simulink model "fresh_control_system"  (R2020a)
settings: Solver=VariableStepAuto  StartTime=0.0  StopTime=7  RelTol=1e-3
libraries: simulink x2, dspfdesign x1
settings Model: Creator=parthmahendru  LastModifiedBy=Mohamed
settings OptimizationCC: DefaultParameterBehavior=Inlined  EnhancedBackFolding=on  PassReuseOutputArgsAs=Individual arguments  ZeroExternalMemoryAtStartup=off  ZeroInternalMemoryAtStartup=off  OptimizeBlockOrder=speed  DifferentSizesBufferReuse=on  EfficientTunableParamExpr=on
settings DebuggingCC: ParameterTunabilityLossMsg=error
settings SFSimCC: MATLABDynamicMemAlloc=off
settings RTWCC: SystemTargetFile=ert.tlc  GenCodeOnly=on  TemplateMakefile=ert_default_tmf
settings CodeAppCC: ForceParamTrailComments=on  IgnoreCustomStorageClasses=off  OperatorAnnotations=on  SimulinkDataObjDesc=on  SFDataObjDesc=on  InsertBlockDesc=on
settings ERTTargetCC: TargetLangStandard=C99 (ISO)  GenerateSampleERTMain=on  InlinedParameterPlacement=NonHierarchical  ERTCustomFileTemplate=example_file_process.tlc

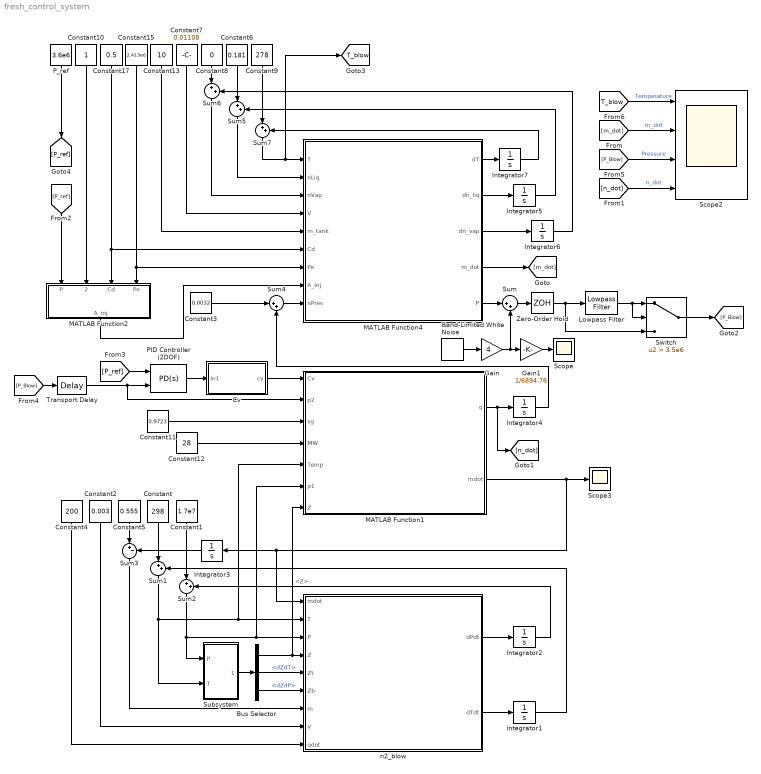
== system fresh_control_system ==
  Band-Limited White Noise : simulink/Sources/Band-Limited White Noise  Cov=100000  Ts=0.001  seed=[23341]
  Bus Selector : BusSelector  OutputSignals=Z,dZdT,dZdP
  Constant : Constant  Value=298
  Constant1 : Constant  Value=1.7e7
  Constant10 : Constant
  Constant11 : Constant  Value=0.9723
  Constant12 : Constant  Value=28
  Constant13 : Constant  Value=10
  Constant15 : Constant  Value=2.413e6  VectorParams1D=off
  Constant17 : Constant  Value=0.5
  Constant2 : Constant  Value=0.003
  Constant3 : Constant  Value=0.0032
  Constant4 : Constant  Value=200
  Constant5 : Constant  Value=0.555
  Constant6 : Constant  Value=0.181
  Constant7 : Constant  Value=0.01108
  Constant8 : Constant  Value=0
  Constant9 : Constant  Value=278
  Cv : Subsystem
  Gain : Gain  Gain=4
  Gain1 : Gain  Gain=1/6894.76
  Integrator{1..7} (7 alike) : Integrator
  Lowpass Filter : dspfdesign/Lowpass Filter  FilterType=FIR  DesignForMinimumOrder=off  FilterOrder=10  PassbandFrequency=700  StopbandFrequency=3000  PassbandRipple=0.1  StopbandAttenuation=80  InheritSampleRate=off  SampleRate=44100  SimulateUsing=Interpreted execution  roundingMode=Nearest  coeffsDataTypeStr=fixdt(1,16)
  MATLAB Function1 : MATLAB Function  TreatAsAtomicUnit=on
  MATLAB Function2 : MATLAB Function  TreatAsAtomicUnit=on
  MATLAB Function4 : MATLAB Function  TreatAsAtomicUnit=on
  PID Controller (2DOF) : simulink/Continuous/PID Controller (2DOF)  Controller=PD  Form=Parallel  TimeDomain=Continuous-time  UseExternalTs=off  SampleTime=-1  IntegratorMethod=Forward Euler  FilterMethod=Forward Euler  ControllerParametersSource=internal  P=3.2e-09  I=1.39281882332403e-13  D=0.9e-05  UseFilter=on  N=1.09398371936337  b=1  c=1  TunerSelectOption=Transfer Function Based (PID Tuner App)  InitialConditionSource=internal  InitialConditionForIntegrator=0  InitialConditionForFilter=0  DifferentiatorICPrevScaledInput=0  ExternalReset=none  TrackingMode=off  Kt=1  LimitOutput=on  UpperSaturationLimit=5  LowerSaturationLimit=0  LinearizeAsGain=on  AntiWindupMode=none  Kb=1  POutMin=[]  POutMax=[]  IOutMin=[]  IOutMax=[]  DOutMin=[]  DOutMax=[]  NOutMin=[]  NOutMax=[]  bOutMin=[]  bOutMax=[]  cOutMin=[]  cOutMax=[]  SumOutMin=[]  SumOutMax=[]  SaturationOutMin=[]  SaturationOutMax=[]  PParamMin=[]  PParamMax=[]  IParamMin=[]  IParamMax=[]  DParamMin=[]  DParamMax=[]  NParamMin=[]  NParamMax=[]  bParamMin=[]  bParamMax=[]  cParamMin=[]  cParamMax=[]  KbParamMin=[]  KbParamMax=[]  KtParamMin=[]  KtParamMax=[]  KbOutMin=[]  KbOutMax=[]  KtOutMin=[]  KtOutMax=[]  IntegratorOutMin=[]  IntegratorOutMax=[]  FilterOutMin=[]  FilterOutMax=[]  SumI1OutMin=[]  SumI1OutMax=[]  SumI2OutMin=[]  SumI2OutMax=[]  SumI3OutMin=[]  SumI3OutMax=[]  SumI4OutMin=[]  SumI4OutMax=[]  SumDOutMin=[]  SumDOutMax=[]  Sum1OutMin=[]  Sum1OutMax=[]  Sum2OutMin=[]  Sum2OutMax=[]  Sum3OutMin=[]  Sum3OutMax=[]  DifferentiatorOutMin=[]  DifferentiatorOutMax=[]  FilterDiffOutCoefMin=[]  FilterDiffOutCoefMax=[]  ReciprocalOutMin=[]  ReciprocalOutMax=[]  SumDenOutMin=[]  SumDenOutMax=[]  SumNumOutMin=[]  SumNumOutMax=[]  DivideOutMin=[]  DivideOutMax=[]  UdiffTsProdOutMin=[]  UdiffTsProdOutMax=[]  NTsProdOutMin=[]  NTsProdOutMax=[]  UintegralTsProdOutMin=[]  UintegralTsProdOutMax=[]  UngainTsProdOutMin=[]  UngainTsProdOutMax=[]  IntegratorContinuousStateAttributes=''  IntegratorStateMustResolveToSignalObject=off  IntegratorRTWStateStorageClass=Auto  FilterContinuousStateAttributes=''  FilterStateMustResolveToSignalObject=off  FilterRTWStateStorageClass=Auto  ParallelPVariant=InternalParameters  IdealPVariant=Disabled  IVariant=Disabled  DVariant=InternalParameters  bVariant=InternalParameters  cVariant=InternalParameters  IntegratorVariant=Disabled  SatVariant=Enabled  AWVariant=Disabled  PCopyVariant=Disabled  TRVariant=Disabled  FdbkBlocksVariant=Forward  IdealPFdbkVariant=Disabled  SatFdbkVariant=Disabled  DerivativeFilterVariant=ContFilter  NVariant=InternalParameters  NCopyVariant=Disabled  FilterICVariant=InternalICsFilter  IntegratorICVariant=Disabled  ExternalResetVariant=Disabled  TRSumVariant=Passthrough  SumFdbkVariant=Disabled  SumVariant=Sum_PD  TsampFilterVariant=InternalTs  TsampNgainVariant=Passthrough  TsampIntegralVariant=Disabled_SignalSpec
  P_ref : Constant  Value=3.6e6
  Scope : Scope
  Scope2 : Scope  NumInputPorts=4
  Scope3 : Scope
  Subsystem : Subsystem
  Sum{,1..2,4..7} (7 alike) : Sum  Inputs=|++
  Sum3 : Sum  Inputs=|+-
  Switch : Switch  Criteria=u2 > Threshold  Threshold=3.5e6
  Transport Delay : TransportDelay  DelayTime=0.01
  Zero-Order Hold : ZeroOrderHold  SampleTime=-1
  n2_blow : MATLAB Function  TreatAsAtomicUnit=on
  tag scope: T_blow=global
  wires:
  PID Controller (2DOF)/1 -> Cv/1(In1)
  MATLAB Function4/4(m_dot) -> [m_dot]
  [m_dot] -> Scope2/2  "m_dot"
  [n_dot] -> Scope2/4  "n_dot"
  [P_Blow] -> Scope2/3  "Pressure"
  [T_blow] -> Scope2/1  "Temperature"
  Constant4/1 -> n2_blow/9(qdot)
  Constant2/1 -> n2_blow/8(V)
  Constant1/1 -> Sum2/1
  n2_blow/1(dPdt) -> Integrator2/1
  Integrator2/1 -> Sum2/2
  Integrator1/1 -> Sum1/2
  n2_blow/2(dTdt) -> Integrator1/1
  Constant/1 -> Sum1/1
  Constant5/1 -> Sum3/1
  Sum3/1 -> n2_blow/7(m)
  MATLAB Function1/2(mdot) -> Scope3/1, n2_blow/1(mdot), Integrator3/1
  Integrator3/1 -> Sum3/2
  Sum4/1 -> MATLAB Function4/9(nPres)
  Constant3/1 -> Sum4/1
  Constant6/1 -> Sum5/1
  MATLAB Function4/1(dT) -> Integrator7/1
  MATLAB Function4/2(dn_liq) -> Integrator5/1
  MATLAB Function4/3(dn_vap) -> Integrator6/1
  Sum5/1 -> MATLAB Function4/2(nLiq)
  Integrator5/1 -> Sum5/2
  Constant8/1 -> Sum6/1
  Sum6/1 -> MATLAB Function4/3(nVap)
  Integrator6/1 -> Sum6/2
  Constant9/1 -> Sum7/1
  Integrator7/1 -> Sum7/2
  Sum7/1 -> [T_blow], MATLAB Function4/1(T)
  MATLAB Function1/1(q) -> [n_dot], Integrator4/1
  Integrator4/1 -> Sum4/2
  Constant7/1 -> MATLAB Function4/4(V)
  Constant13/1 -> MATLAB Function4/5(m_tank)
  Constant15/1 -> MATLAB Function2/4(Pe), MATLAB Function4/7(Pe)
  Constant17/1 -> MATLAB Function2/3(Cd), MATLAB Function4/6(Cd)
  MATLAB Function2/1(A_inj) -> MATLAB Function4/8(A_inj)
  Constant10/1 -> MATLAB Function2/2(m_dot_des)
  P_ref/1 -> [P_ref]
  [P_ref] -> MATLAB Function2/1(P)
  MATLAB Function4/5(P) -> Sum/1
  Band-Limited White Noise/1 -> Gain/1
  [P_ref] -> PID Controller (2DOF)/1
  [P_Blow] -> Transport Delay/1
  Sum/1 -> Zero-Order Hold/1
  Zero-Order Hold/1 -> Lowpass Filter/1, Switch/3
  Gain/1 -> Sum/2, Gain1/1
  Switch/1 -> [P_Blow]
  Lowpass Filter/1 -> Switch/2, Switch/1
  Gain1/1 -> Scope/1
  Sum2/1 -> MATLAB Function1/6(p1), n2_blow/3(P), Subsystem/1(P)
  Sum1/1 -> MATLAB Function1/5(Temp), n2_blow/2(T), Subsystem/2(T)
  Subsystem/1(Outport) -> Bus Selector/1
  Bus Selector/2 -> n2_blow/5(Zt)  "<dZdT>"
  Bus Selector/3 -> n2_blow/6(Zb)  "<dZdP>"
  Bus Selector/1 -> MATLAB Function1/7(Z), n2_blow/4(Z)  "<Z>"
  Constant11/1 -> MATLAB Function1/3(sg)
  Constant12/1 -> MATLAB Function1/4(MW)
  Transport Delay/1 -> MATLAB Function1/2(p2), PID Controller (2DOF)/2
  Cv/1(cv) -> MATLAB Function1/1(Cv)

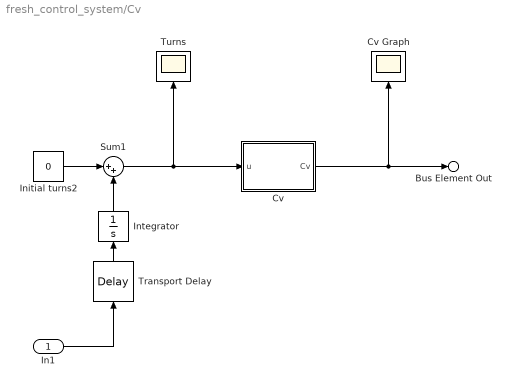
== system fresh_control_system/Cv ==
  In1 : Inport
  Cv : MATLAB Function  TreatAsAtomicUnit=on
  Cv Graph : Scope
  Initial turns2 : Constant  Value=0
  Integrator : Integrator
  Sum1 : Sum  Inputs=|++
  Transport Delay : TransportDelay  DelayTime=0.004
  Turns : Scope
  Bus Element Out : Outport  PortName=cv  Element=signal1
  wires:
  In1/1 -> Transport Delay/1
  Integrator/1 -> Sum1/2
  Initial turns2/1 -> Sum1/1
  Cv/1(Cv) -> Cv Graph/1, Bus Element Out/1
  Sum1/1 -> Cv/1(u), Turns/1
  Transport Delay/1 -> Integrator/1

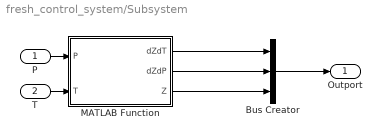
== system fresh_control_system/Subsystem ==
  P : Inport
  T : Inport  Port=2
  Bus Creator : BusCreator  Inputs=3
  MATLAB Function : MATLAB Function  TreatAsAtomicUnit=on
  Outport : Outport
  wires:
  MATLAB Function/1(dZdT) -> Bus Creator/1
  T/1 -> MATLAB Function/2(T)
  MATLAB Function/2(dZdP) -> Bus Creator/2
  P/1 -> MATLAB Function/1(P)
  MATLAB Function/3(Z) -> Bus Creator/3
  Bus Creator/1 -> Outport/1

== matlab function fresh_control_system/MATLAB Function2 ==
  data: P input; A_inj output; m_dot_des input; Cd input; Pe input
function A_inj  = A_inj(P, m_dot_des, Cd, Pe)
MW=44;
Vhat_l=0.05;

A_inj=(m_dot_des)/(Cd*sqrt(abs(2/MW*(P - Pe)/Vhat_l))*MW);

== matlab function fresh_control_system/n2_blow ==
  data: mdot input; T input; P input; Z input; Zt input; Zb input; m input; V input; dPdt output; qdot input; dTdt output
function [dPdt, dTdt] = n2_blowdown(mdot, T, P, Z, Zt, Zb, m, V, qdot)

    R = 8314 / 28;
    cnv = 6894.76;

    Zp = Zb/cnv;
    cv = 776;

    dPdt = (m*R*Z^2 + P*V*Zt)*qdot/(V*cv*(m*(Z - P*Zp)))    ...
         - mdot*((cv + Z*R)*m*Z + P*V*Zt)*(P/(m*cv))/(m*(Z - P*Zp));

    dZdt = (m*R*Z^2 * Zp + V*Z*Zt)*dPdt/(m*R*Z^2 + P*V)     ...
         - Zt*(P*V*Z/m)*mdot/(m*R*Z^2 + P*V);

    dTdt = V*(dPdt/(m*Z) - dZdt*P/(m*Z^2) - mdot*P/(m*Z^2))/R;
end

== matlab function fresh_control_system/Subsystem/MATLAB Function ==
  data: P input; T input; dZdT output; dZdP output; Z output
function [dZdT, dZdP, Z]  = get_dZ_N2(P, T)

    P           = P / 6894.76;
    
    nh_theta    = [0.90370032155133;...
                          -3.99164830787538;...
                           4.44554878990612;...
                          -1.68387394930366;...
                           1.84282855081908;...
                          -2.71807522455834;...
                           1.80658523674363;...
                          -0.00026662830718;...
                           0.16405364316350];

    nh_alpha    = [1;               ...
                           0.45607085009281;...
                           0.99224794564113;...
                           1.58495789262624;...
                           0.53133147588636;...
                           1.29132167947510;...
                           1.44008913900161;...
                           2.74997487910292;...
                           2.36611999082672];

    nl_theta    = [0.46742656471647;...
                          -0.53799565472298;...
                          -9.22454428760102;...
                           9.15603503101003;...
                           3.18808664459882;...
                           0.30163700042055;...
                          -0.27300234680706;...
                          -1.00749719408221;...
                          -1.49106816983329];

    nl_alpha    = [1;               ...
                           1.41102397459172;...
                           0.33562799290636;...
                           0.79810083070486;...
                           0.01008992455881;...
                           2.53968667359886;...
                           2.51281397715323;...
                           1.20879498088509;...
                           1.69572064361084];
                       
    if (T >= 220 && T <= 320) && (P >= 800 && P <= 4500)

        T           = T / 126.2;
        P           = P / 492.3;

        dZdTr       = nh_theta(2)*nh_alpha(2)*T^(nh_alpha(2) - 1)*P^0.7   ...
                    + nh_theta(3)*nh_alpha(3)*T^(nh_alpha(3) - 1)*P^0.5   ...
                    + nh_theta(4)*nh_alpha(4)*T^(nh_alpha(4) - 1)*P^0.3   ...
                    + nh_theta(5)*nh_alpha(5)*T^(nh_alpha(5) - 1)*P       ...
                    + nh_theta(6)*nh_alpha(6)*T^(nh_alpha(6) - 1)*P       ...
                    + nh_theta(7)*nh_alpha(7)*T^(nh_alpha(7) - 1)*P       ...
                    + nh_theta(9)*nh_alpha(9)*T^(nh_alpha(9) - 1);

        dZdT        = dZdTr / 126.2;

        dZdPr       = 0.7*nh_theta(2)*T^nh_alpha(2)*P^(-0.3)        ...
                    + 0.5*nh_theta(3)*T^nh_alpha(3)*P^(-0.5)        ...
                    + 0.3*nh_theta(4)*T^nh_alpha(4)*P^(-0.7)        ...
                    + nh_theta(5)*T^nh_alpha(5)                     ...
                    + nh_theta(6)*T^nh_alpha(6)                     ...
                    + nh_theta(7)*T^nh_alpha(7)                     ...
                    + nh_theta(8)*nh_alpha(8)*P^(nh_alpha(8) - 1);

        dZdP        = dZdPr / 492.3;     

        N           = [1;                       ...
                        T^nh_alpha(2)*P^0.7;     ...
                        T^nh_alpha(3)*P^0.5;     ...
                        T^nh_alpha(4)*P^0.3;     ...
                        T^nh_alpha(5)*P;           ...
                        T^nh_alpha(6)*P;           ...
                        T^nh_alpha(7)*P;           ...
                        P^nh_alpha(8);             ...
                        T^nh_alpha(9)];               

        Z       = sum(nh_theta .* N);        

    elseif (T >= 180 && T < 220) && (P >= 800 && P <= 4500)

        T           = T / 126.2;
        P           = P / 492.3;

        dZdTr       = nl_theta(2)*nl_alpha(2)*T^(nl_alpha(2) - 1)*P^0.7   ...
                    + nl_theta(3)*nl_alpha(3)*T^(nl_alpha(3) - 1)*P^0.5   ...
                    + nl_theta(4)*nl_alpha(4)*T^(nl_alpha(4) - 1)*P^0.3   ...
                    + nl_theta(5)*nl_alpha(5)*T^(nl_alpha(5) - 1)*P       ...
                    + nl_theta(6)*nl_alpha(6)*T^(nl_alpha(6) - 1)*P       ...
                    + nl_theta(7)*nl_alpha(7)*T^(nl_alpha(7) - 1)*P       ...
                    + nl_theta(9)*nl_alpha(9)*T^(nl_alpha(9) - 1);

        dZdT        = dZdTr / 126.2;

        dZdPr       = 0.7*nl_theta(2)*T^nl_alpha(2)*P^(-0.3)        ...
                    + 0.5*nl_theta(3)*T^nl_alpha(3)*P^(-0.5)        ...
                    + 0.3*nl_theta(4)*T^nl_alpha(4)*P^(-0.7)        ...
                    + nl_theta(5)*T^nl_alpha(5)                     ...
                    + nl_theta(6)*T^nl_alpha(6)                     ...
                    + nl_theta(7)*T^nl_alpha(7)                     ...
                    + nl_theta(8)*nl_alpha(8)*P^(nl_alpha(8) - 1);

        dZdP        = dZdPr / 492.3;     

        N           = [1;                       ...
                        T^nl_alpha(2)*P^0.7;     ...
                        T^nl_alpha(3)*P^0.5;     ...
                        T^nl_alpha(4)*P^0.3;     ...
                        T^nl_alpha(5)*P;           ...
                        T^nl_alpha(6)*P;           ...
                        T^nl_alpha(7)*P;           ...
                        P^nl_alpha(8);             ...
                        T^nl_alpha(9)];               

        Z       = sum(nl_theta .* N); 

    else
        T           = 180 / 126.2;
        P           = P / 492.3;

        dZdTr       = nl_theta(2)*nl_alpha(2)*T^(nl_alpha(2) - 1)*P^0.7   ...
                    + nl_theta(3)*nl_alpha(3)*T^(nl_alpha(3) - 1)*P^0.5   ...
                    + nl_theta(4)*nl_alpha(4)*T^(nl_alpha(4) - 1)*P^0.3   ...
                    + nl_theta(5)*nl_alpha(5)*T^(nl_alpha(5) - 1)*P       ...
                    + nl_theta(6)*nl_alpha(6)*T^(nl_alpha(6) - 1)*P       ...
                    + nl_theta(7)*nl_alpha(7)*T^(nl_alpha(7) - 1)*P       ...
                    + nl_theta(9)*nl_alpha(9)*T^(nl_alpha(9) - 1);

        dZdT        = dZdTr / 126.2;

        dZdPr       = 0.7*nl_theta(2)*T^nl_alpha(2)*P^(-0.3)        ...
                    + 0.5*nl_theta(3)*T^nl_alpha(3)*P^(-0.5)        ...
                    + 0.3*nl_theta(4)*T^nl_alpha(4)*P^(-0.7)        ...
                    + nl_theta(5)*T^nl_alpha(5)                     ...
                    + nl_theta(6)*T^nl_alpha(6)                     ...
                    + nl_theta(7)*T^nl_alpha(7)                     ...
                    + nl_theta(8)*nl_alpha(8)*P^(nl_alpha(8) - 1);

        dZdP        = dZdPr / 492.3;  

    N           = [1;                       ...
                    T^nl_alpha(2)*P^0.7;     ...
                    T^nl_alpha(3)*P^0.5;     ...
                    T^nl_alpha(4)*P^0.3;     ...
                    T^nl_alpha(5)*P;           ...
                    T^nl_alpha(6)*P;           ...
                    T^nl_alpha(7)*P;           ...
                    P^nl_alpha(8);             ...
                    T^nl_alpha(9)];               

    Z       = sum(nl_theta .* N); 

    end
end

== matlab function fresh_control_system/MATLAB Function4 ==
  data: T input; dT output; dn_liq output; dn_vap output; m_dot output; nLiq input; nVap input; V input; m_tank input; Cd input; Pe input; A_inj input; P output; nPres input
function [dT, dn_liq, dn_vap, m_dot, P] = nox_blowdown(T, nLiq, nVap, V, m_tank, Cd, Pe, A_inj, nPres )
%OX_TANK_SIM Models thermochemical processes of blow-down in oxidizer tank.
%   Propellant Tank Pressurization Modeling for a Hybrid Rocket - Margaret
%   Mary Fernandez
%
%   INPUTS:
%       "n" = 1x2 vector of ox moles in tank (kmol).
%       "T" = ox tank temperature (K).
%       "V" = volume of ox tank (m^3).
%       "m_tank" = mass of oxidizer tank (kg).
%       "m_dot_prev" = ox mass flow rate of previous time step (kg/s).
%       "A_inj" = total orifice area of injector plate (m^2).
%       "Cd" = injector plate discharge coefficient.
%       "Pe" = pressure at exit of injector plate (Pa).
%
%   OUTPUTS:
%       "m_dot" = scalar ox mass flow rate (kg/s).
%       "dn" = 1x2 differential change in ox moles (kmol).
%       "dT" = differential change in ox tank temperature (K).
%       "P" = scalar internal pressure of ox tank (Pa).
%%%%%%%%%%%%%%%%%%%%%%%%%%%%%%%%%%%%%%%%%%%%%%%%%%%%%%%%%%%%%%%%%%%%%%%%%%%

%Perry's Chemical Engineers' Handbook Property Equations:
G1 = 96.512;           %Vapour pressure of N2O [Pa] coefficients
G2 = -4045;            % valid for Temp range [182.3 K - 309.57 K]
G3 = -12.277;
G4 = 2.886e-5;
G5 = 2;

Tc = 309.57;           % critical temperature of N2O [K]

J1 = 2.3215e7;         % heat of vaporization of N2O [J/kmol] coefficients
J2 = 0.384;            % valid for Temp range [182.3 K - 309.57 K]
J3 = 0;
J4 = 0;

% % heat capacity of N2 at constant pressure [J/(kmol*K)] coefficients
% % valid for Temp range [100 K - 1500 K]
% C1 = 0.28883e5; 
% C2 = 0;              
% C3 = 0;
% C4 = 0;
% C5 = 0;

D1 = 0.2934e5; % heat capacity of N2O gas at constant pressure [J/(kmol*K)] coefficients
D2 = 0.3236e5; % valid for Temp range [100 K - 1500 K]
D3 = 1.1238e3;
D4 = 0.2177e5;
D5 = 479.4; 

E1 = 6.7556e4; % heat capacity of N2O liquid at constant pressure [J/(kmol*K)] coefficients
E2 = 5.4373e1; % valid for Temp range [182.3 K - 200 K]
E3 = 0;
E4 = 0;
E5 = 0;
Q1 = 2.781;    % molar specific volume of liquid N2O [m^3/kmol] coefficients
Q2 = 0.27244;
Q3 = 309.57;
Q4 = 0.2882;

R  = 8314;      %Universal gas constant (J/kmol*K).
MW = 44.013;   %Molar mass of N2O (kg/kmol)​
% Calculate thermodynamic parameters as functions of temperature:
Vhat_l      = Q2^(1 + (1 - T/Q3)^Q4)/Q1;                    %Molar specific vol. of liq. N2O [m^3/kmol]
CVhat_g     = D1 + D2*((D3/T)/sinh(D3/T))^2 + ...
              D4*((D5/T)/cosh(D5/T))^2 - R;                 %Molar c_V of N2O gas [J/(kmol*K)]
CVhat_l     = E1 + E2*T + E3*T^2 + E4*T^3 + E5*T^4;         %Molar c_V of N2O liq.; approx. = c_P [J/(kmol*K)]
Tr          = T/Tc;                                         %Reduced temperature.
delta_Hv    = J1*(1 - Tr) ^ (J2 + J3*Tr + J4*Tr^2);         %Heat of vaporization of N2O [J/kmol]
P_sat       = exp(G1 + G2/T + G3*log(T) + G4*T^G5);         %Vapour P of N20 (Pa).
dP_sat      = (-G2/(T^2) + G3/T + G4*G5*T^(G5-1)) ...       %Derivative of vapour P with respect to T.
              * exp(G1 + G2/T + G3*log(T) + G4*T^G5);        
c_P         = (4.8 + 0.00322*T)*155.239;                    %Specific heat of tank, Aluminum [J/kg*K]


%Simplified expression definitions for solution:
P = (nPres+nVap)*R*T/(V - nLiq*Vhat_l);
a = m_tank*c_P  + nPres*CVhat_l+nVap*CVhat_g + nLiq*CVhat_l;
RT = P*Vhat_l;
e = -delta_Hv + R*T;
f = -Cd*A_inj*sqrt(abs(2/MW*(P - Pe)/Vhat_l));
j = -Vhat_l*P_sat;
k = (V - nLiq*Vhat_l)*dP_sat;
l = R*T;
q = R*nVap;
Z = (-f*(-j*a + (q - k)*RT))/(a*(l + j) + (q - k)*(e - RT));
W = (-Z*(l*a + (q - k)*e))/(-j*a + (q - k)*RT);
%Time derivative of tank conditions
m_dot = -f*MW;          % Mass flow rate
dn_liq    = W;    % Time derivative of nitrous amount
dn_vap=Z;
dT    = (RT*W + e*Z)/a;  % Time derivative of tank temperature

end

== matlab function fresh_control_system/Cv/Cv ==
  data: Cv output; u input
function Cv = Cvcalc(u)
Cv = u/20;

% if (u<2)
%     Cv = u/20;
% % elseif(u>6&&u<9)
% % Cv=((1.1169*(u-5.95)^2))/100+0.03;
% else
%   Cv=0;
%     
% end
% 
%     
% % till 0.1
end

== matlab function fresh_control_system/MATLAB Function1 ==
  data: Cv input; p2 input; sg input; MW input; Temp input; p1 input; q output; mdot output; Z input
function [q, mdot]   = Needle_valve(Cv,p2,sg,MW,Temp,p1,Z)
    %sg is specific gravity
    
    p1_new=p1/98066.5;
    p2_new=p2/98066.5;

    del_p=p1_new-p2_new;
    
    R = 8314 / 28;
    rho = p1 / (R * Z * Temp);

    if (p2>0.5*p1)
        q=0.11362272*Cv*p1_new*(1-(2*del_p)/(3*p1_new))*sqrt((del_p/(p1_new*sg*Temp)))* rho/MW * (101325/p1 * Temp/288);
        mdot=q*MW;
    else
        q=0.471*0.11362272*Cv*p1_new*sqrt(1/(sg*Temp)) * rho/MW * (101325/p1 * Temp/288);
        mdot=q*MW;
    end

end
